simulink model "Control_LQR_Model_Simulink_2"  (R2021a)
settings: Solver=VariableStepAuto  StartTime=0.0  StopTime=25  RelTol=1e-3
values from neighbouring files (symbols this model uses):
  A = []    [Fixed_Model.m]    (also in Matlab_Linear_Model.m = [0 1 ; 0 -Br/I]; Matlab__Linear_Model.m = [0 1 ; 0 Br/I]; Matlab__Linear_Model_2.m = [0 1 ; 0 -Br/I]; Matlab__NonLinear_Model.m = [0 1 ; 0 Br/I])
  B = []    [Fixed_Model.m]    (also in Matlab_Linear_Model.m = [0 ;1]; Matlab__Linear_Model.m = [0 0 ; 1/I -l2x/I]; Matlab__Linear_Model_2.m = [B(:,2)]; Matlab__NonLinear_Model.m = [0 0 ; -H/I -l2x/I])
  C = [1 0]    [Matlab_Linear_Model.m]    (also in Matlab__Linear_Model.m; Matlab__Linear_Model_2.m = [1 1]; Matlab__NonLinear_Model.m; Mc1.mat)
  g = 9.81    [Fixed_Model.m]    (also in Matlab_Linear_Model.m; Matlab__Linear_Model.m; Matlab__Linear_Model_2.m; Matlab__NonLinear_Model.m)
  K = lqr(A,B,Q,R)    [Matlab_Linear_Model.m]    (also in Matlab__Linear_Model.m; Matlab__Linear_Model_2.m; Mc1.mat = [1 0.446480452821]; initialize.m)
  l2f = (l1 + l2)/2 + l3f + l3o    (= 0.65)    [Matlab_Linear_Model.m]    (also in Matlab__Linear_Model_2.m; Mc1.mat; initialize.m; jsp.m)
  l3f = l3o + 0.15    (= 0.3)    [Matlab_Linear_Model.m]    (also in Matlab__Linear_Model.m; Matlab__Linear_Model_2.m; Matlab__NonLinear_Model.m; Mc1.mat)
  l3o = 0.3    [Fixed_Model.m]    (also in Matlab_Linear_Model.m = 0.15; Matlab__Linear_Model.m = 0.15; Matlab__Linear_Model_2.m = 0.15; Matlab__NonLinear_Model.m = 0.15)
  m2 = 2    [Fixed_Model.m]    (also in Matlab_Linear_Model.m = 1.4; Matlab__Linear_Model.m; Matlab__Linear_Model_2.m; Matlab__NonLinear_Model.m = 1.5)
  x0 = [pi/8;0]    [Matlab_Linear_Model.m]    (also in Matlab__Linear_Model.m = [pi/2;0]; Matlab__Linear_Model_2.m = [pi/2;0]; Matlab__NonLinear_Model.m = [pi/2;0]; Mc1.mat = [1.57079632679 0])
undefined symbols (not defined in the file or in its folder): DiscIntNeverNeededParam
libraries: simulink x6
settings Model: Creator=DANI-TUF  LastModifiedBy=DANI-TUF

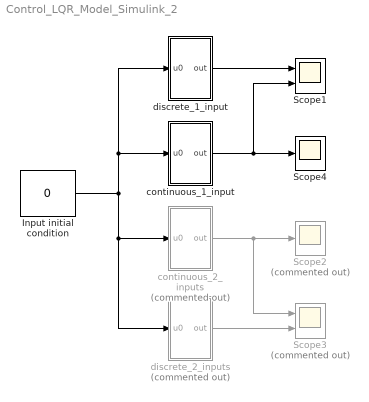
== system Control_LQR_Model_Simulink_2 ==
  Input initial condition : Constant  Value=0
  Scope1 : Scope  NumInputPorts=2
  Scope2 : Scope  Commented=on
  Scope3 : Scope  Commented=on  NumInputPorts=2
  Scope4 : Scope
  continuous_1_input : Subsystem
  continuous_2_inputs : Subsystem  Commented=on
  discrete_1_input : Subsystem
  discrete_2_inputs : Subsystem  Commented=on
  wires:
  continuous_2_inputs/1(out) -> Scope3/1, Scope2/1
  discrete_2_inputs/1(out) -> Scope3/2
  continuous_1_input/1(out) -> Scope1/2, Scope4/1
  discrete_1_input/1(out) -> Scope1/1
  Input initial condition/1 -> continuous_2_inputs/1(u0), discrete_2_inputs/1(u0), discrete_1_input/1(u0), continuous_1_input/1(u0)

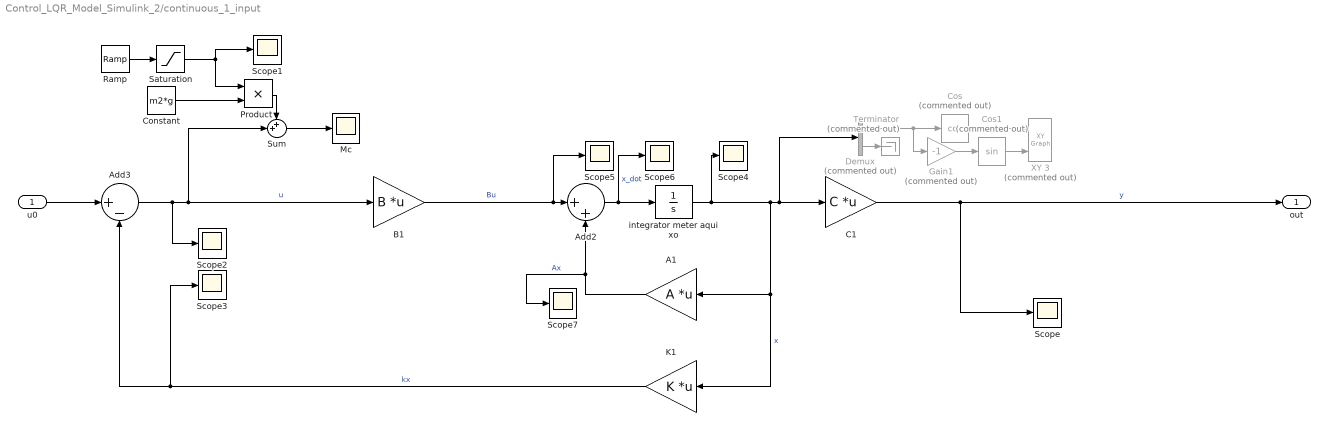
== system Control_LQR_Model_Simulink_2/continuous_1_input ==
  u0 : Inport
  A1 : Gain  Gain=A  Multiplication=Matrix(K*u)
  Add2 : Sum  Inputs=|++
  Add3 : Sum  Inputs=|+-
  B1 : Gain  Gain=B  Multiplication=Matrix(K*u)
  C1 : Gain  Gain=C  Multiplication=Matrix(K*u)
  Constant : Constant  Value=m2*g
  Cos : Trigonometry  Commented=on  Operator=cos
  Cos1 : Trigonometry  Commented=on
  Demux : Demux  Commented=on  Outputs=2
  Gain1 : Gain  Commented=on  Gain=-1
  K1 : Gain  Gain=K  Multiplication=Matrix(K*u)
  Mc : Scope
  Product : Product
  Ramp : simulink/Sources/Ramp  slope=0.025  start=5  InitialOutput=l2f+l3o-l3f
  Saturation : Saturate  UpperLimit=l2f
  Scope{,1..7} (8 alike) : Scope
  Sum : Sum  Inputs=++|
  Terminator : Terminator  Commented=on
  XY 3 : simulink/Sinks/XY Graph  Commented=on  xmin=-2  xmax=2  ymin=-2  ymax=2  st=-1
  integrator meter aqui xo : Integrator  InitialCondition=x0
  out : Outport
  wires:
  Demux/2 -> Terminator/1
  C1/1 -> Scope/1, out/1  "y"
  Cos/1 -> XY 3/1
  Cos1/1 -> XY 3/2
  A1/1 -> Add2/2, Scope7/1  "Ax"
  u0/1 -> Add3/1
  B1/1 -> Add2/1, Scope5/1  "Bu"
  integrator meter aqui xo/1 -> A1/1, K1/1, Demux/1, C1/1, Scope4/1  "x"
  Add2/1 -> integrator meter aqui xo/1, Scope6/1  "x_dot"
  K1/1 -> Scope3/1, Add3/2  "kx"
  Add3/1 -> Scope2/1, Sum/2, B1/1  "u"
  Gain1/1 -> Cos1/1
  Demux/1 -> Gain1/1, Cos/1
  Sum/1 -> Mc/1
  Constant/1 -> Product/2
  Ramp/1 -> Saturation/1
  Saturation/1 -> Product/1, Scope1/1
  Product/1 -> Sum/1

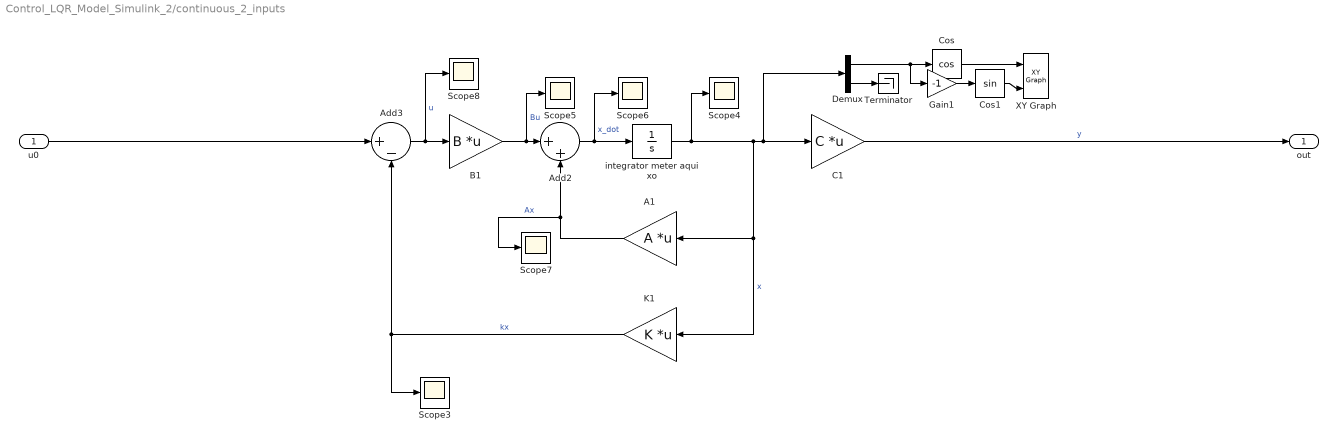
== system Control_LQR_Model_Simulink_2/continuous_2_inputs ==
  u0 : Inport
  A1 : Gain  Gain=A  Multiplication=Matrix(K*u)
  Add2 : Sum  Inputs=|++
  Add3 : Sum  Inputs=|+-
  B1 : Gain  Gain=B  Multiplication=Matrix(K*u)
  C1 : Gain  Gain=C  Multiplication=Matrix(K*u)
  Cos : Trigonometry  Operator=cos
  Cos1 : Trigonometry
  Demux : Demux  Outputs=2
  Gain1 : Gain  Gain=-1
  K1 : Gain  Gain=K  Multiplication=Matrix(K*u)
  Scope{3..8} (6 alike) : Scope
  Terminator : Terminator
  XY Graph : simulink/Sinks/XY Graph  xmin=-2  xmax=2  ymin=-2  ymax=2  st=-1
  integrator meter aqui xo : Integrator  InitialCondition=[pi/16; 0]
  out : Outport
  wires:
  K1/1 -> Add3/2, Scope3/1  "kx"
  Add2/1 -> Scope6/1, integrator meter aqui xo/1  "x_dot"
  Demux/1 -> Gain1/1, Cos/1
  integrator meter aqui xo/1 -> Scope4/1, Demux/1, C1/1, K1/1, A1/1  "x"
  B1/1 -> Scope5/1, Add2/1  "Bu"
  Add3/1 -> Scope8/1, B1/1  "u"
  u0/1 -> Add3/1
  A1/1 -> Scope7/1, Add2/2  "Ax"
  Cos1/1 -> XY Graph/2
  Cos/1 -> XY Graph/1
  C1/1 -> out/1  "y"
  Demux/2 -> Terminator/1
  Gain1/1 -> Cos1/1

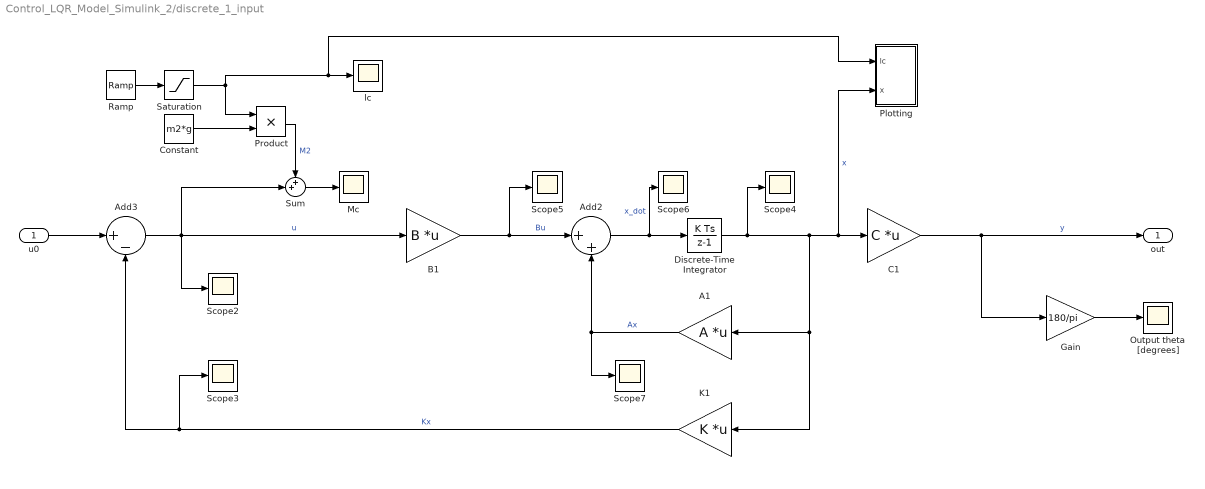
== system Control_LQR_Model_Simulink_2/discrete_1_input ==
  u0 : Inport
  A1 : Gain  Gain=A  Multiplication=Matrix(K*u)
  Add2 : Sum  Inputs=|++
  Add3 : Sum  Inputs=|+-
  B1 : Gain  Gain=B  Multiplication=Matrix(K*u)
  C1 : Gain  Gain=C  Multiplication=Matrix(K*u)
  Constant : Constant  Value=m2*g
  Discrete-Time Integrator : DiscreteIntegrator  InitialCondition=x0  SampleTime=1e-3  ICPrevOutput=DiscIntNeverNeededParam  ICPrevScaledInput=DiscIntNeverNeededParam
  Gain : Gain  Gain=180/pi
  K1 : Gain  Gain=K  Multiplication=Matrix(K*u)
  Mc : Scope
  Output theta [degrees] : Scope
  Plotting : Subsystem
  Product : Product
  Ramp : simulink/Sources/Ramp  slope=0.025  start=5  InitialOutput=l2f+l3o-l3f
  Saturation : Saturate  UpperLimit=l2f
  Scope{2..7} (6 alike) : Scope
  Sum : Sum  Inputs=++|
  lc : Scope
  out : Outport
  wires:
  Product/1 -> Sum/1  "M2"
  Saturation/1 -> Plotting/1(lc), lc/1, Product/1
  Ramp/1 -> Saturation/1
  Constant/1 -> Product/2
  Sum/1 -> Mc/1
  Add3/1 -> B1/1, Sum/2, Scope2/1  "u"
  K1/1 -> Add3/2, Scope3/1  "Kx"
  Add2/1 -> Discrete-Time Integrator/1, Scope6/1  "x_dot"
  Discrete-Time Integrator/1 -> Scope4/1, Plotting/2(x), C1/1, K1/1, A1/1  "x"
  B1/1 -> Add2/1, Scope5/1  "Bu"
  u0/1 -> Add3/1
  A1/1 -> Add2/2, Scope7/1  "Ax"
  C1/1 -> out/1, Gain/1  "y"
  Gain/1 -> Output theta [degrees]/1

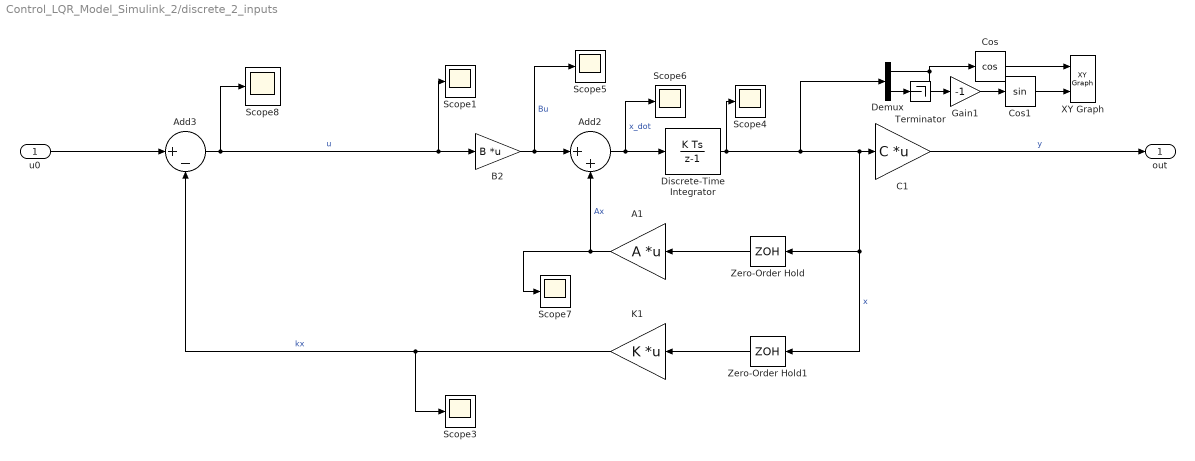
== system Control_LQR_Model_Simulink_2/discrete_2_inputs ==
  u0 : Inport
  A1 : Gain  Gain=A  Multiplication=Matrix(K*u)
  Add2 : Sum  Inputs=|++
  Add3 : Sum  Inputs=|+-
  B2 : Gain  Gain=B  Multiplication=Matrix(K*u)
  C1 : Gain  Gain=C  Multiplication=Matrix(K*u)
  Cos : Trigonometry  Operator=cos
  Cos1 : Trigonometry
  Demux : Demux  Outputs=2
  Discrete-Time Integrator : DiscreteIntegrator  InitialCondition=[pi/16 ;0]  SampleTime=1e-3  ICPrevOutput=DiscIntNeverNeededParam  ICPrevScaledInput=DiscIntNeverNeededParam
  Gain1 : Gain  Gain=-1
  K1 : Gain  Gain=K  Multiplication=Matrix(K*u)
  Scope{1,3..8} (7 alike) : Scope
  Terminator : Terminator
  XY Graph : simulink/Sinks/XY Graph  xmin=-2  xmax=2  ymin=-2  ymax=2  st=-1
  Zero-Order Hold : ZeroOrderHold  SampleTime=1e-3
  Zero-Order Hold1 : ZeroOrderHold  SampleTime=1e-3
  out : Outport
  wires:
  Demux/2 -> Terminator/1
  C1/1 -> out/1  "y"
  Cos/1 -> XY Graph/1
  Cos1/1 -> XY Graph/2
  A1/1 -> Add2/2, Scope7/1  "Ax"
  u0/1 -> Add3/1
  Add3/1 -> Scope1/1, B2/1, Scope8/1  "u"
  Discrete-Time Integrator/1 -> Demux/1, Zero-Order Hold/1, Zero-Order Hold1/1, C1/1, Scope4/1  "x"
  Demux/1 -> Cos/1, Gain1/1
  Add2/1 -> Discrete-Time Integrator/1, Scope6/1  "x_dot"
  K1/1 -> Scope3/1, Add3/2  "kx"
  Zero-Order Hold/1 -> A1/1
  Zero-Order Hold1/1 -> K1/1
  B2/1 -> Scope5/1, Add2/1  "Bu"
  Gain1/1 -> Cos1/1

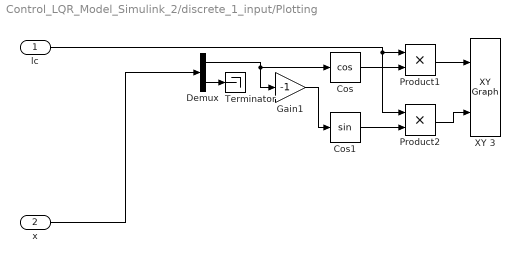
== system Control_LQR_Model_Simulink_2/discrete_1_input/Plotting ==
  lc : Inport
  x : Inport  Port=2
  Cos : Trigonometry  Operator=cos
  Cos1 : Trigonometry
  Demux : Demux  Outputs=2
  Gain1 : Gain  Gain=-1
  Product1 : Product
  Product2 : Product
  Terminator : Terminator
  XY 3 : simulink/Sinks/XY Graph  xmin=-1  xmax=1.5  ymin=-1  ymax=1.5  st=-1
  wires:
  Demux/2 -> Terminator/1
  Cos/1 -> Product1/2
  Demux/1 -> Cos/1, Gain1/1
  Product2/1 -> XY 3/2
  Cos1/1 -> Product2/2
  lc/1 -> Product2/1, Product1/1
  Gain1/1 -> Cos1/1
  Product1/1 -> XY 3/1
  x/1 -> Demux/1
